simulink model "chuaSMC_sim"  (R2024a)
settings: Solver=VariableStepAuto  StartTime=0.0  StopTime=t_sim  RelTol=1e-3
settings Model: Creator=lorenzo  LastModifiedBy=lorenzo

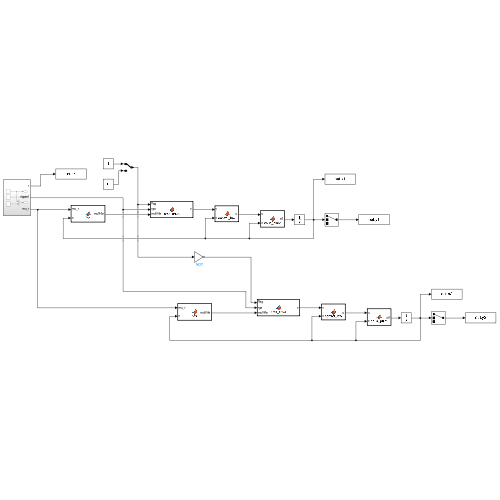
[thumbnail: Simulink's stored preview of the top-level diagram]
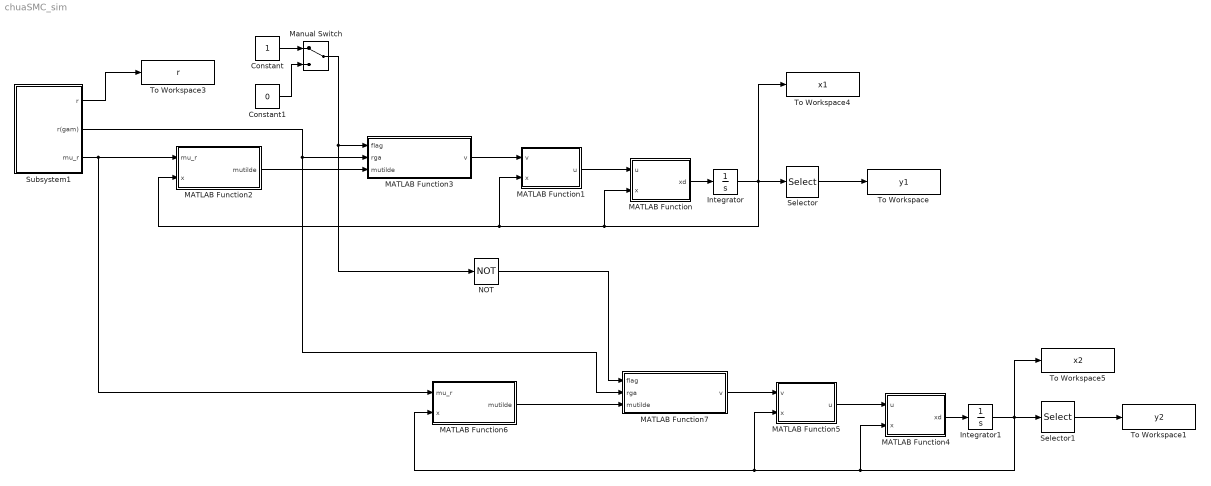
== system chuaSMC_sim ==
  Constant : Constant
  Constant1 : Constant  Value=0
  Integrator : Integrator
  Integrator1 : Integrator
  MATLAB Function : MATLAB Function  TreatAsAtomicUnit=on
  MATLAB Function1 : MATLAB Function  TreatAsAtomicUnit=on
  MATLAB Function2 : MATLAB Function  TreatAsAtomicUnit=on
  MATLAB Function3 : MATLAB Function  TreatAsAtomicUnit=on
  MATLAB Function4 : MATLAB Function  TreatAsAtomicUnit=on
  MATLAB Function5 : MATLAB Function  TreatAsAtomicUnit=on
  MATLAB Function6 : MATLAB Function  TreatAsAtomicUnit=on
  MATLAB Function7 : MATLAB Function  TreatAsAtomicUnit=on
  Manual Switch : ManualSwitch
  NOT : Logic  Operator=NOT  IconShape=distinctive  AllPortsSameDT=off  OutDataTypeStr=boolean
  Selector : Selector  InputPortWidth=3  IndexOptions=Index vector (dialog)  Indices=1  OutputSizes=1
  Selector1 : Selector  InputPortWidth=3  IndexOptions=Index vector (dialog)  Indices=1  OutputSizes=1
  Subsystem1 : Subsystem
  To Workspace : ToWorkspace  VariableName=y1  SaveFormat=Timeseries  SampleTime=-1
  To Workspace1 : ToWorkspace  VariableName=y2  SaveFormat=Timeseries  SampleTime=-1
  To Workspace3 : ToWorkspace  VariableName=r  SaveFormat=Timeseries  SampleTime=-1
  To Workspace4 : ToWorkspace  VariableName=x1  SaveFormat=Timeseries  SampleTime=-1
  To Workspace5 : ToWorkspace  VariableName=x2  SaveFormat=Timeseries  SampleTime=-1
  wires:
  MATLAB Function/1(xd) -> Integrator/1
  Integrator/1 -> To Workspace4/1, Selector/1, MATLAB Function1/2(x), MATLAB Function2/2(x), MATLAB Function/2(x)
  MATLAB Function1/1(u) -> MATLAB Function/1(u)
  MATLAB Function2/1(mutilde) -> MATLAB Function3/3(mutilde)
  MATLAB Function3/1(v) -> MATLAB Function1/1(v)
  Subsystem1/3(mu_r) -> MATLAB Function2/1(mu_r), MATLAB Function6/1(mu_r)
  Selector/1 -> To Workspace/1
  Subsystem1/2(r(gam)) -> MATLAB Function3/2(rga), MATLAB Function7/2(rga)
  Constant/1 -> Manual Switch/1
  Constant1/1 -> Manual Switch/2
  Manual Switch/1 -> NOT/1, MATLAB Function3/1(flag)
  Subsystem1/1(r) -> To Workspace3/1
  MATLAB Function7/1(v) -> MATLAB Function5/1(v)
  Selector1/1 -> To Workspace1/1
  MATLAB Function6/1(mutilde) -> MATLAB Function7/3(mutilde)
  MATLAB Function5/1(u) -> MATLAB Function4/1(u)
  MATLAB Function4/1(xd) -> Integrator1/1
  Integrator1/1 -> To Workspace5/1, Selector1/1, MATLAB Function5/2(x), MATLAB Function6/2(x), MATLAB Function4/2(x)
  NOT/1 -> MATLAB Function7/1(flag)

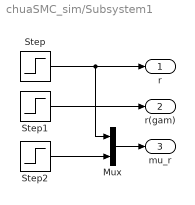
== system chuaSMC_sim/Subsystem1 ==
  Mux : Mux  Inputs=2
  Step : Step  Time=0  SampleTime=0
  Step1 : Step  Time=0  After=0  SampleTime=0
  Step2 : Step  Time=0  After=0  SampleTime=0
  r : Outport  VectorParamsAs1DForOutWhenUnconnected=off
  r(gam) : Outport  Port=2  VectorParamsAs1DForOutWhenUnconnected=off
  mu_r : Outport  Port=3  VectorParamsAs1DForOutWhenUnconnected=off
  wires:
  Step/1 -> Mux/1, r/1
  Step1/1 -> r(gam)/1
  Step2/1 -> Mux/2
  Mux/1 -> mu_r/1

== matlab function chuaSMC_sim/MATLAB Function1 ==
  data: v input; u output; x input
function u = control_law(v,x)

alpha = 10.4;

rho_hat = -1.194*x(1) + 0.0422*x(1)^3;
rho_hatd = (633*x(1)^2)/5000 - 597/500; 

u = v/alpha - (x(1)-x(2)+x(3)-alpha*(x(2)-x(1)-rho_hat)*(1+rho_hatd));

== matlab function chuaSMC_sim/MATLAB Function ==
  data: u input; xd output; x input
function xd = chua_plant(u,x)

R = 0.1; alpha = 10.4; beta = 16.5;
rho = -1.16*x(1) + 0.041*x(1)^3;

xd = [alpha*(x(2)-x(1)-rho);
 x(1)-x(2)+x(3)+u;
 -beta*x(2)-R*x(3)];

== matlab function chuaSMC_sim/MATLAB Function2 ==
  data: mu_r input; x input; mutilde output
function mutilde = fcn(mu_r,x)

alpha = 10.4;
rho_hat = -1.194*x(1) + 0.0422*x(1)^3;
mu = [x(1); alpha*(x(2)-x(1)-rho_hat)];


mutilde = mu_r - mu;

== matlab function chuaSMC_sim/MATLAB Function4 ==
  data: u input; xd output; x input
function xd = chua_plant(u,x)

R = 0.1; alpha = 10.4; beta = 16.5;
rho = -1.16*x(1) + 0.041*x(1)^3;

xd = [alpha*(x(2)-x(1)-rho);
 x(1)-x(2)+x(3)+u;
 -beta*x(2)-R*x(3)];

== matlab function chuaSMC_sim/MATLAB Function3 ==
  data: flag input; rga input; v output; mutilde input
function v=smc_chua(flag,rga,mutilde)

% parameters
k1=50;
k2=40;

if flag

    eta=0.5;
    
    % sliding surface function
    s=mutilde(2)+k2*mutilde(1);
    
    % sliding mode control law
    v=rga+k2*mutilde(2)+k1*sign(s);
    % v=rga+k2*mutilde(2)+k1*tanh(eta*s);

else

    % feedback linearization control law
    v=rga+k2*mutilde(2)+k1*mutilde(1);

end

== matlab function chuaSMC_sim/MATLAB Function5 ==
  data: v input; u output; x input
function u = control_law(v,x)

alpha = 10.4;

rho_hat = -1.194*x(1) + 0.0422*x(1)^3;
rho_hatd = (633*x(1)^2)/5000 - 597/500; 

u = v/alpha - (x(1)-x(2)+x(3)-alpha*(x(2)-x(1)-rho_hat)*(1+rho_hatd));

== matlab function chuaSMC_sim/MATLAB Function6 ==
  data: mu_r input; x input; mutilde output
function mutilde = fcn(mu_r,x)

alpha = 10.4;
rho_hat = -1.194*x(1) + 0.0422*x(1)^3;
mu = [x(1); alpha*(x(2)-x(1)-rho_hat)];


mutilde = mu_r - mu;

== matlab function chuaSMC_sim/MATLAB Function7 ==
  data: flag input; rga input; v output; mutilde input
function v=smc_chua(flag,rga,mutilde)

% parameters
k1=50;
k2=30;

if flag

    eta=0.5;
    
    % sliding surface function
    s=mutilde(2)+k2*mutilde(1);
    
    % sliding mode control law
    % v=rga+k2*mutilde(2)+k1*sign(s);
    v=rga+k2*mutilde(2)+k1*tanh(eta*s);

else

    % feedback linearization control law
    v=rga+k2*mutilde(2)+k1*mutilde(1);

end
